simulink model "eCS_Algo_Simulation"  (R2018a)
settings: Solver=ode1  StartTime=0.0  StopTime=0.2  FixedStep=1/80000  RelTol=1e-3  EnableMultiTasking=on
PostLoadFcn:
  | , if any(exist('dsrtsu_mdlpostloadfcn', 'file') == [2, 3, 6]), try dsrtsu_mdlpostloadfcn('Execute', bdroot); catch fprintf('Error in PostLoadFcn (dsrtsu_mdlpostloadfcn) for model "%s":\n %s\n', bdroot, lasterr); end, end,
values from neighbouring files (symbols this model uses):
  AccSensor = 5    [Parameter_eCS_Algo.m]
  AlgoType = 0    [Parameter_eCS_Algo.m]
  Cxy = 1*0.017    (= 0.017)    [Acc_Init_SelV1.m]
  Cxz = 1*0.017    (= 0.017)    [Acc_Init_SelV1.m]
  Cyx = 1*0.017    (= 0.017)    [Acc_Init_SelV1.m]
  Cyz = 1*0.017    (= 0.017)    [Acc_Init_SelV1.m]
  Czx = 1*0.017    (= 0.017)    [Acc_Init_SelV1.m]
  Czy = 1*0.017    (= 0.017)    [Acc_Init_SelV1.m]
  FreqTemperature = 10    [Acc_Init_SelV1.m]
  MaxSensorOffset = 0.3    [Acc_Init_SelV1.m]
  Mean_x_noise = 4e-3    (= 0.004)    [Acc_Init_SelV1.m]
  Mean_y_noise = 4e-3    (= 0.004)    [Acc_Init_SelV1.m]
  Mean_z_noise = 4e-3    (= 0.004)    [Acc_Init_SelV1.m]
  ODR = 8000    [Acc_Init_SelV1.m]
  offsetcorrection_on_off = 0    [Parameter_eCS_Algo.m]
  pulsetype = 2    [Parameter_eCS_Algo.m]    (also in run_simulation.m = j; run_simulation_ActiveX.m = j)
  Range = 4    [Acc_Init_SelV1.m]
  TempBias = 0    [Acc_Init_SelV1.m]
  TemperatureAmp = 0    [Acc_Init_SelV1.m]
  Var_x_noise = 1.84e-9    (= 1.84e-09)    [Acc_Init_SelV1.m]
  Var_y_noise = 2.025e-09    [Acc_Init_SelV1.m]
  Var_z_noise = 1.374e-09    [Acc_Init_SelV1.m]
  w_x = 2*pi*F_x    (= 376.991118431)    [Acc_Init_SelV1.m]
  w_y = 2*pi*F_y    (= 376.991118431)    [Acc_Init_SelV1.m]
  w_z = 2*pi*F_z    (= 376.991118431)    [Acc_Init_SelV1.m]
  x_max_temp_drift = 0.061    [Acc_Init_SelV1.m]
  x_offset_enable = 0    [Acc_Init_SelV1.m]
  x_run_to_run_drift = 0.0    (= 0)    [Acc_Init_SelV1.m]
  x_temp_co_drift = 0.000    (= 0)    [Acc_Init_SelV1.m]
  Xi_x = 0.7    [Acc_Init_SelV1.m]
  Xi_y = 0.7    [Acc_Init_SelV1.m]
  Xi_z = 0.7    [Acc_Init_SelV1.m]
  y_max_temp_drift = 0.061    [Acc_Init_SelV1.m]
  y_offset_enable = 0    [Acc_Init_SelV1.m]
  y_run_to_run_drift = 0.0    (= 0)    [Acc_Init_SelV1.m]
  y_temp_co_drift = 0.000    (= 0)    [Acc_Init_SelV1.m]
  z_max_temp_drift = 0.13    [Acc_Init_SelV1.m]
  z_offset_enable = 0    [Acc_Init_SelV1.m]
  z_run_to_run_drift = 0.0    (= 0)    [Acc_Init_SelV1.m]
  z_temp_co_drift = 0.000    (= 0)    [Acc_Init_SelV1.m]
undefined symbols (not defined in the file or in its folder): controller_sample_rate, DiscIntNeverNeededParam, gmw_roada_x__m_s__, gmw_roada_y__m_s__, gmw_roadtime_2kHz, Meldorf_HindenburgstraAcceleration_x__m_s_2_, Meldorf_HindenburgstraAcceleration_y__m_s_2_, Meldorf_HindenburgstraTime__s_, pulse_FF27, pulse_MPDB, pulse_ODB40, pulse_ODB64, pulse_USNCAP, pulsetime_FF27, pulsetime_MPDB, pulsetime_ODB40, pulsetime_ODB64, pulsetime_USNCAP, sigbuilder_block, VW_416_2kHza_x_2kHz, VW_416_2kHza_y_2kHz, VW_416_2kHztime_2kHz
libraries: simulink x23, dspsigops x1
(part 2 of 2)

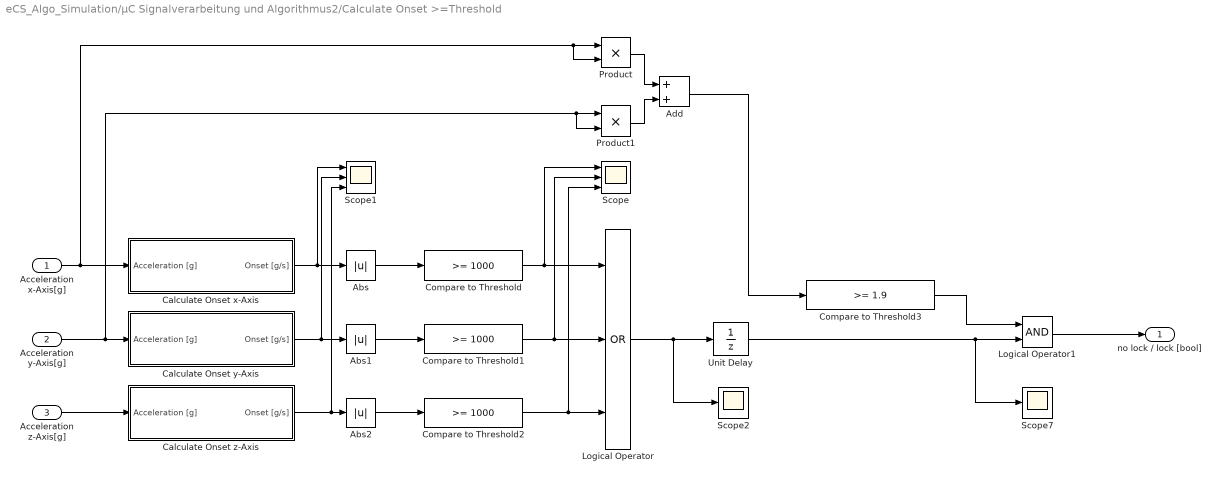
== system eCS_Algo_Simulation/µC Signalverarbeitung und Algorithmus2/Calculate Onset >=Threshold ==
  Acceleration x-Axis[g] : Inport
  Acceleration y-Axis[g] : Inport  Port=2
  Acceleration z-Axis[g] : Inport  Port=3
  Abs : Abs
  Abs1 : Abs
  Abs2 : Abs
  Add : Sum
  Calculate Onset x-Axis : Subsystem
  Calculate Onset y-Axis : Subsystem
  Calculate Onset z-Axis : Subsystem
  Compare to Threshold : simulink/Logic and Bit Operations/Compare To Constant  relop=>=  const=1000  OutDataTypeStr=boolean
  Compare to Threshold1 : simulink/Logic and Bit Operations/Compare To Constant  relop=>=  const=1000  OutDataTypeStr=boolean
  Compare to Threshold2 : simulink/Logic and Bit Operations/Compare To Constant  relop=>=  const=1000  OutDataTypeStr=boolean
  Compare to Threshold3 : simulink/Logic and Bit Operations/Compare To Constant  relop=>=  const=1.9  OutDataTypeStr=boolean
  Logical Operator : Logic  Operator=OR  Inputs=3  AllPortsSameDT=off  OutDataTypeStr=boolean
  Logical Operator1 : Logic  AllPortsSameDT=off  OutDataTypeStr=boolean
  Product : Product
  Product1 : Product
  Scope : Scope  NumInputPorts=3
  Scope1 : Scope  NumInputPorts=3
  Scope2 : Scope
  Scope7 : Scope
  Unit Delay : UnitDelay  SampleTime=1/1000
  no lock / lock [bool] : Outport
  wires:
  Product1/1 -> Add/2
  Compare to Threshold3/1 -> Logical Operator1/1
  Add/1 -> Compare to Threshold3/1
  Acceleration y-Axis[g]/1 -> Product1/2, Product1/1, Calculate Onset y-Axis/1(Acceleration [g])
  Calculate Onset x-Axis/1(Onset [g/s]) -> Scope1/1, Abs/1
  Compare to Threshold1/1 -> Scope/2, Logical Operator/2
  Acceleration x-Axis[g]/1 -> Product/2, Product/1, Calculate Onset x-Axis/1(Acceleration [g])
  Product/1 -> Add/1
  Compare to Threshold/1 -> Scope/1, Logical Operator/1
  Logical Operator1/1 -> no lock / lock [bool]/1
  Abs1/1 -> Compare to Threshold1/1
  Calculate Onset y-Axis/1(Onset [g/s]) -> Scope1/2, Abs1/1
  Abs2/1 -> Compare to Threshold2/1
  Logical Operator/1 -> Scope2/1, Unit Delay/1
  Compare to Threshold2/1 -> Scope/3, Logical Operator/3
  Acceleration z-Axis[g]/1 -> Calculate Onset z-Axis/1(Acceleration [g])
  Unit Delay/1 -> Scope7/1, Logical Operator1/2
  Abs/1 -> Compare to Threshold/1
  Calculate Onset z-Axis/1(Onset [g/s]) -> Scope1/3, Abs2/1

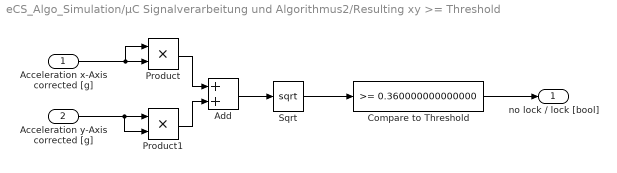
== system eCS_Algo_Simulation/µC Signalverarbeitung und Algorithmus2/Resulting xy >= Threshold ==
  Acceleration x-Axis corrected [g] : Inport
  Acceleration y-Axis corrected [g] : Inport  Port=2
  Add : Sum
  Compare to Threshold : simulink/Logic and Bit Operations/Compare To Constant  relop=>=  const=0.360000000000000  OutDataTypeStr=boolean
  Product : Product
  Product1 : Product
  Sqrt : Sqrt  SaturateOnIntegerOverflow=on
  no lock / lock [bool] : Outport
  wires:
  Compare to Threshold/1 -> no lock / lock [bool]/1
  Sqrt/1 -> Compare to Threshold/1
  Product/1 -> Add/1
  Product1/1 -> Add/2
  Add/1 -> Sqrt/1
  Acceleration x-Axis corrected [g]/1 -> Product/2, Product/1
  Acceleration y-Axis corrected [g]/1 -> Product1/1, Product1/2

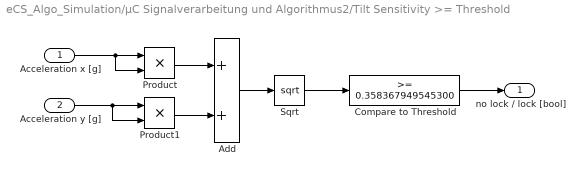
== system eCS_Algo_Simulation/µC Signalverarbeitung und Algorithmus2/Tilt Sensitivity >= Threshold ==
  Acceleration x [g] : Inport
  Acceleration y [g] : Inport  Port=2
  Add : Sum
  Compare to Threshold : simulink/Logic and Bit Operations/Compare To Constant  relop=>=  const=0.358367949545300  OutDataTypeStr=boolean
  Product : Product
  Product1 : Product
  Sqrt : Sqrt  SaturateOnIntegerOverflow=on
  no lock / lock [bool] : Outport
  wires:
  Sqrt/1 -> Compare to Threshold/1
  Product/1 -> Add/1
  Add/1 -> Sqrt/1
  Compare to Threshold/1 -> no lock / lock [bool]/1
  Acceleration x [g]/1 -> Product/2, Product/1
  Acceleration y [g]/1 -> Product1/2, Product1/1
  Product1/1 -> Add/2

== system eCS_Algo_Simulation/µC Signalverarbeitung und Algorithmus2/Calculate Onset >=Threshold/Calculate Onset x-Axis ==
  Acceleration [g] : Inport
  Detect Change : simulink/Logic and Bit Operations/Detect Change  vinit=0  OutDataTypeStr=boolean
  Faktor2 : SampleTimeMath  TsampMathOp=/  TsampMathImp=Offline Scaling Adjustment
  Gain : Gain  Gain=10000/100000
  Triggered Subsystem : Subsystem  TreatAsAtomicUnit=on
  delta x : Sum  Inputs=+-
  Onset [g/s] : Outport
  wires:
  Gain/1 -> Onset [g/s]/1
  Faktor2/1 -> Triggered Subsystem/1(In), Detect Change/1, delta x/1
  Detect Change/1 -> Triggered Subsystem/Trigger
  Triggered Subsystem/1(Out1) -> delta x/2
  delta x/1 -> Gain/1
  Acceleration [g]/1 -> Faktor2/1

== system eCS_Algo_Simulation/µC Signalverarbeitung und Algorithmus2/Calculate Onset >=Threshold/Calculate Onset y-Axis ==
  Acceleration [g] : Inport
  Detect Change : simulink/Logic and Bit Operations/Detect Change  vinit=0  OutDataTypeStr=boolean
  Faktor2 : SampleTimeMath  TsampMathOp=/  TsampMathImp=Offline Scaling Adjustment
  Gain : Gain  Gain=10000/100000
  Triggered Subsystem : Subsystem  TreatAsAtomicUnit=on
  delta x : Sum  Inputs=+-
  Onset [g/s] : Outport
  wires:
  Acceleration [g]/1 -> Faktor2/1
  delta x/1 -> Gain/1
  Triggered Subsystem/1(Out1) -> delta x/2
  Detect Change/1 -> Triggered Subsystem/Trigger
  Faktor2/1 -> Triggered Subsystem/1(In), delta x/1, Detect Change/1
  Gain/1 -> Onset [g/s]/1

== system eCS_Algo_Simulation/µC Signalverarbeitung und Algorithmus2/Calculate Onset >=Threshold/Calculate Onset z-Axis ==
  Acceleration [g] : Inport
  Detect Change : simulink/Logic and Bit Operations/Detect Change  vinit=0  OutDataTypeStr=boolean
  Faktor2 : SampleTimeMath  TsampMathOp=/  TsampMathImp=Offline Scaling Adjustment
  Gain : Gain  Gain=10000/100000
  Sample and Hold : dspsigops/Sample and Hold  Commented=on  trig=Rising edge  initCond=-controller_sample_rate  latchinput=on
  Triggered Subsystem : Subsystem  TreatAsAtomicUnit=on
  delta x : Sum  Inputs=+-
  Onset [g/s] : Outport
  wires:
  Gain/1 -> Onset [g/s]/1
  Faktor2/1 -> Triggered Subsystem/1(In), Detect Change/1, delta x/1
  Detect Change/1 -> Triggered Subsystem/Trigger
  Triggered Subsystem/1(Out1) -> delta x/2
  delta x/1 -> Gain/1
  Acceleration [g]/1 -> Faktor2/1

== system eCS_Algo_Simulation/µC Signalverarbeitung und Algorithmus2/Calculate Onset >=Threshold/Calculate Onset x-Axis/Triggered Subsystem ==
  In : Inport  LatchByDelayingOutsideSignal=on
  Trigger : TriggerPort  VariantControl=Variant
  Out1 : Outport
  wires:
  In/1 -> Out1/1

== system eCS_Algo_Simulation/µC Signalverarbeitung und Algorithmus2/Calculate Onset >=Threshold/Calculate Onset y-Axis/Triggered Subsystem ==
  In : Inport  LatchByDelayingOutsideSignal=on
  Trigger : TriggerPort  VariantControl=Variant
  Out1 : Outport
  wires:
  In/1 -> Out1/1

== system eCS_Algo_Simulation/µC Signalverarbeitung und Algorithmus2/Calculate Onset >=Threshold/Calculate Onset z-Axis/Triggered Subsystem ==
  In : Inport  LatchByDelayingOutsideSignal=on
  Trigger : TriggerPort  VariantControl=Variant
  Out1 : Outport
  wires:
  In/1 -> Out1/1

== matlab function eCS_Algo_Simulation/retractor locking trigger ==
  settings: updateMethod=DISCRETE
  data: trigger_solenoid input; s input; s_mech_locking input; trigger_retractor output; time input; triggertime_retractor output; s_locking output
function [trigger_retractor,triggertime_retractor,s_locking]     = retractor_locking_trigger(trigger_solenoid, s, s_mech_locking,time)

%local variable declaration
persistent s_store
persistent trigger_old
persistent trigger_intern
persistent t_store
persistent s_locking_intern
persistent once

% Initialisation
if isempty(s_store)
    s_store=10000;
    trigger_old=0;
    trigger_intern=0;    
    t_store=0;
    s_locking_intern=0;
    once=0;
end


%main
if and(trigger_old==0, trigger_solenoid==1)
    trigger_old=1;
    s_store=s;
    %s_locking_intern=s;
end

if and(s-s_store>s_mech_locking , once==0)
    once=1;
    trigger_intern=1;
    t_store=time;
    s_locking_intern=s;
end

% Output 
trigger_retractor=trigger_intern;
triggertime_retractor=t_store * 1000;
s_locking=s_locking_intern;

== matlab function eCS_Algo_Simulation/trigger travels, times and counts ==
  settings: updateMethod=DISCRETE
  data: s_locking output; trigger input; s input; triggertime output; time input; triggercounts output
function [s_locking , triggertime, triggercounts]     = triggertime(trigger , s , time)
%Input a trigger signal (0 to 1)n and calculate/output the triggertime in ms
%local variable declaration
persistent trigger_once
persistent triggertime_intern
persistent s_locking_intern
persistent triggercounts_intern
persistent trigger_old

% Initialisation
if isempty(trigger_once)
   trigger_once=0;
   triggertime_intern = 0 ;
   s_locking_intern = 0 ;   
   triggercounts_intern = 0 ;
   trigger_old=0;   
end


%main

    %one-time detection of first trigger to set triggertime and travel
    if and (trigger_once==0 , trigger==1)
        trigger_once=1;
        triggertime_intern=time*1000;
        s_locking_intern = s ;  
    end

    %count the number of triggers
    if trigger_old~=trigger
        trigger_old=trigger;
        triggercounts_intern=triggercounts_intern+0.5;
    end    
    
    
% Output 
triggertime=triggertime_intern;
s_locking=s_locking_intern;
triggercounts=triggercounts_intern;

== matlab function eCS_Algo_Simulation/trigger travels, times and counts1 ==
  settings: updateMethod=DISCRETE
  data: s_locking output; trigger input; s input; triggertime output; time input; triggercounts output
function [s_locking , triggertime, triggercounts]     = triggertime(trigger , s , time)
%Input a trigger signal (0 to 1)n and calculate/output the triggertime in ms
%local variable declaration
persistent trigger_once
persistent triggertime_intern
persistent s_locking_intern
persistent triggercounts_intern
persistent trigger_old

% Initialisation
if isempty(trigger_once)
   trigger_once=0;
   triggertime_intern = 0 ;
   s_locking_intern = 0 ;   
   triggercounts_intern = 0 ;
   trigger_old=0;   
end


%main

    %one-time detection of first trigger to set triggertime and travel
    if and (trigger_once==0 , trigger==1)
        trigger_once=1;
        triggertime_intern=time*1000;
        s_locking_intern = s ;  
    end

    %count the number of triggers
    if trigger_old~=trigger
        trigger_old=trigger;
        triggercounts_intern=triggercounts_intern+0.5;
    end    
    
    
% Output 
triggertime=triggertime_intern;
s_locking=s_locking_intern;
triggercounts=triggercounts_intern;

== matlab function eCS_Algo_Simulation/eCS Algo new/aceleration clipping trigger ==
  settings: updateMethod=DISCRETE
  data: trigger_out output; pulse_in input; triggertime output; time input; no_of_samples input; a_threshold input
function [trigger_out , triggertime]     = acceleration_clipping_trigger(pulse_in, time, no_of_samples, a_threshold)
%Inputthe pulse signal and count the number of subsequent samples above the
%acceleration threshold - when the numer of allowed samples are reached,
%then the trigger_out goes from 1 to 0 for a certain hold-time
%intention is to detect a crahs-pulse a.s.a.p when the acceleration signal
%excceeds a certain threshold

%local variable declaration
persistent trigger_intern
persistent triggertime_intern
persistent samples_counter


% Initialisation
if isempty(trigger_intern)
   trigger_intern=0;
   triggertime_intern = 0 ;
   samples_counter = 0 ;   
end


%main
if pulse_in>=a_threshold
    samples_counter = samples_counter+1 ;
else
    samples_counter=0;
end



if  and( samples_counter>=no_of_samples , trigger_intern==0)
    trigger_intern=1;
    triggertime_intern=time*1000;
end

if and ( and( samples_counter<no_of_samples , trigger_intern==1) , (time-(triggertime_intern/1000)) > 0.1 )
    trigger_intern=0;
end
% Output
trigger_out=trigger_intern;
triggertime=triggertime_intern;

== matlab function eCS_Algo_Simulation/eCS Algo new/Trigger_hold_time ==
  data: trigger_in input; trigger_out output; time input; time_delay input
function trigger_out    = Trigger_hold_time(trigger_in,time,time_delay)
%no impact on trigger change from 0 to 1 (-->locking)
%delays the time for the trigger signal from 1 to 0 (-->unlocking) to avoid
%too many subsequent locking in a certain time

%local variable declaration
persistent time_store
persistent trigger_intern

% Initialisation
if isempty(time_store)
   time_store = 0 ;
   trigger_intern = 0 ;   
end

% main
if trigger_in==1 ;
    time_store=time;
    trigger_intern=trigger_in;
end
if time>=(time_store+ (time_delay/1000) );
    trigger_intern=trigger_in;
end

% Output
trigger_out=trigger_intern;

== matlab function eCS_Algo_Simulation/solenoid time delay ==
  settings: updateMethod=DISCRETE
  data: trigger input; trigger_out output; time input; dt_to_lock input; dt_to_unlock input
function trigger_out     = solenoid_time_delay(trigger,time,dt_to_lock,dt_to_unlock)

%local variable declaration
persistent trigger_old
persistent trigger_intern
persistent t_on
persistent t_off


% Initialisation
if isempty(trigger_old)
   trigger_old=0;
   trigger_intern = 0 ;   
   t_on=-1;      %delay time for switching on
   t_off=-1;      %delay time for switching off   
end


%main
if and (trigger_old==0 , trigger==1)
    trigger_old=1;
    t_on=time;
    t_off=-1;
end
if and (trigger_old==1 , trigger==0)
    trigger_old=0;
    t_off=time;
    t_on=-1;    
end

if and ( time-t_on>=dt_to_lock/1000 , time-t_on<1)
       trigger_intern=1; 
end    
if and ( time-t_off>=dt_to_unlock/1000 , time-t_off<1)
       trigger_intern=0; 
end   

% Output 
trigger_out=trigger_intern;
